simulink model "clamped_plate_NASTRAN_aug"  (R2025b)
settings: Solver=VariableStepAuto  StartTime=0.0  StopTime=10  RelTol=1e-3
libraries: RCTblocks x1
settings Model: Creator=f.sanfedino  LastModifiedBy=andre
settings SolverCC: AlgebraicLoopSolver=TrustRegion
settings DataIOCC: ReturnWorkspaceOutputs=off
settings DebuggingCC: UnconnectedInputMsg=warning  UnconnectedOutputMsg=warning  UnconnectedLineMsg=warning
settings ModelReferenceCC: EnableRefExpFcnMdlSchedulingChecks=on
settings RTWCC: GPUComputeCapability=3.5  DLArmComputeVersion=19.05

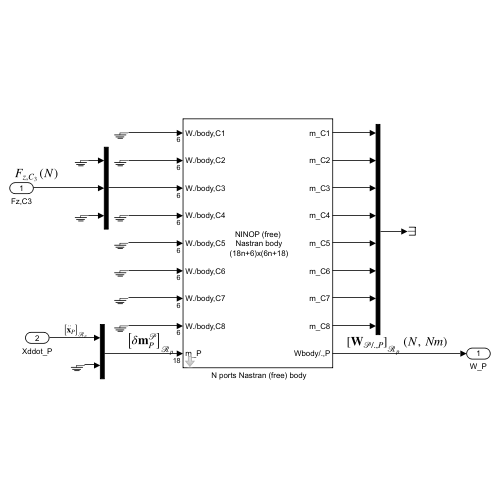
[thumbnail: Simulink's stored preview of the top-level diagram]
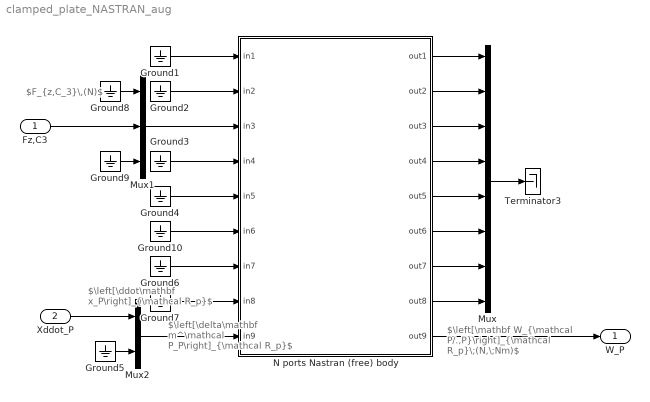
== system clamped_plate_NASTRAN_aug ==
  note: $F_{z,C_3}\,(N)$
  note: $\left[\mathbf W_{\mathcal P/.,P}\right]_{\mathcal R_p}\;(N,\;Nm)$
  note: $\left[\delta\mathbf m^\mathcal P_P\right]_{\mathcal R_p}$
  note: $\left[\ddot\mathbf x_P\right]_{\mathcal R_p}$
  Fz,C3 : Inport
  Xddot_P : Inport  Port=2
  " N ports Nastran (free) body" : Subsystem  mask(NINOP Model of a Nastran body){fbdf='fbdf_plate', ff06='ff06_plate', P_gp=56, C_gp=[1;6;11;61;66;111;116;121], nf=20, Xi=0.001, free=off, uw_var=0, Nflex_w=0, uls_var=5, Nflex_LP=0, uev_var=0, Nflex_EV=0}
      mask prompts: fbdf "Name of the .bdf file (without extension)"; ff06 "Name of the .f06 file (without extension)"; P_gp "Node number corresponding to the point P (connection with parent body)"; C_gp "Node numbers corresponding to the points C (connections with child bodies)"; nf "Number of modes to be considered"; Xi "Common damping ratio"; free "Free body at P"; uw_var "uncertainties (%)"; Nflex_w "number of flexible modes (integer)"; uls_var "uncertainties (%)"; Nflex_LP "number of flexible modes (integer)"; uev_var "uncertainties (%)"; Nflex_EV "number of flexible modes (integer)"
      mask help:
      | NINOP (18n+6)x(6n+18) model of a flexible body at points C (connection point with the child  bodies) and point P (connection point with a parent body).
      | * 18nx6n transfer between the wrench applied to this body at the child points C  and motion vectors at these points
      | * 6x18 transfer between the motion vector at the "parent" point P  and the wrench applied by this body at this point
      | The model is expressed In the (inherit) body frame.
      |
      | Model is built from  the data provided by Patran/Nastran analysis output files.
      | Uncertainties can be added to the main parameters.
      |
      | RK: The last channel associated to parent port P can be inverted to free the body at the point P. In that case, 6 rigid modes (12 integrators) are added in the model to output the motion vector at the point P and the model becomes 18(n+1)x6(n+1).
      mask init:
      | n = length(C_gp);
      | NastranBodyNPortAugFree
      mask Help: web('DocNPortNastranBody.html','-browser')
      mask DialogControl Container2 Prompt: Main parameters
      mask DialogControl Container6 Prompt: Parametric uncertainties:
      mask DialogControl Container8 Prompt: Frequencies
      mask DialogControl Control18 Prompt: A common relative uncertainty (%) on the first flexible mode frequencies can be added (uncertainties can be changed later)
      mask DialogControl Control3 Prompt: The uncertain frequency is named: 'w_name_i' where:
      mask DialogControl Control4 Prompt: * 'name' is the current block name (reduced to its alphanumeric characters).
      mask DialogControl Control17 Prompt: * 'i' is the flexible mode number (increasing frequency order)
      mask DialogControl Container9 Prompt: Modal participation factors
      mask DialogControl Control20 Prompt: A common relative uncertainty (%) on the modal participation factors of the first flexible modes can be added (uncertainties can be changed later)
      mask DialogControl Control6 Prompt: The uncertain modal participation factor is named: 'LP_name_iXX' where:
      mask DialogControl Control7 Prompt: *  'name' is the current block name (reduced to its alphanumeric characters),
      mask DialogControl Control8 Prompt: * 'i' is the flexible mode number (increasing frequency order),
      mask DialogControl Control9 Prompt: * 'XX' = 'Tx', 'Ty', 'Tz', 'Rx', 'Ry', 'Rz'.
      mask DialogControl Container10 Prompt: Modal shapes
      mask DialogControl Control21 Prompt: A common relative uncertainty (%) on each eigen vector components at points C for the first flexible modes can be added (uncertainties can be changed later)
      mask DialogControl Control16 Prompt: WARNING: can generate very long process time !!
      mask DialogControl Control11 Prompt: The uncertain component is named: "EV_name_Cj_iXX' where:
      mask DialogControl Control12 Prompt: * 'name' is the current block name (reduced to its alphanumeric characters).
      mask DialogControl Control13 Prompt: * 'j' is the point C number,
      mask DialogControl Control14 Prompt: * 'i' is the flexible mode number (increasing frequency order),
      mask DialogControl Control15 Prompt: * 'XX' = 'Tx', 'Ty', 'Tz', 'Rx', 'Ry', 'Rz'.
      mask Display:
      | if free
      |     disp('NINOP (free)\n Nastran body\n 18(n+1)x6(n+1)')
      | else
      |     disp('NINOP (free)\n Nastran body\n (18n+6)x(6n+18)')
      | end
      | 
      | for ii=1:n
      |         port_label('input', ii,['W./body,C',num2str(ii)])
      |         port_label('output',ii,['m_C',num2str(ii)])
      | end
      | 
      | if free
      |     port_label('input', n+1,'W./body,P')
      |     port_label('output',n+1,'m_P')
      | else
      |     port_label('input', n+1,'m_P')
      |     port_label('output',n+1,'Wbody/.,P')
      | end
  Ground{1..10} (10 alike) : Ground
  Mux : Mux  Inputs=18*ones(1,8)
  Mux1 : Mux  Inputs=[2 1 3]
  Mux2 : Mux  Inputs=[6 12]
  Terminator3 : Terminator
  W_P : Outport
  wires:
  Mux2/1 -> " N ports Nastran (free) body"/9(in9)
  Ground1/1 -> " N ports Nastran (free) body"/1(in1)
  Ground2/1 -> " N ports Nastran (free) body"/2(in2)
  Ground4/1 -> " N ports Nastran (free) body"/5(in5)
  Ground3/1 -> " N ports Nastran (free) body"/4(in4)
  Ground6/1 -> " N ports Nastran (free) body"/7(in7)
  Ground7/1 -> " N ports Nastran (free) body"/8(in8)
  " N ports Nastran (free) body"/1(out1) -> Mux/1
  " N ports Nastran (free) body"/2(out2) -> Mux/2
  " N ports Nastran (free) body"/3(out3) -> Mux/3
  " N ports Nastran (free) body"/4(out4) -> Mux/4
  " N ports Nastran (free) body"/5(out5) -> Mux/5
  " N ports Nastran (free) body"/6(out6) -> Mux/6
  " N ports Nastran (free) body"/7(out7) -> Mux/7
  " N ports Nastran (free) body"/8(out8) -> Mux/8
  " N ports Nastran (free) body"/9(out9) -> W_P/1
  Mux1/1 -> " N ports Nastran (free) body"/3(in3)
  Ground8/1 -> Mux1/1
  Ground9/1 -> Mux1/3
  Ground10/1 -> " N ports Nastran (free) body"/6(in6)
  Fz,C3/1 -> Mux1/2
  Mux/1 -> Terminator3/1
  Xddot_P/1 -> Mux2/1
  Ground5/1 -> Mux2/2

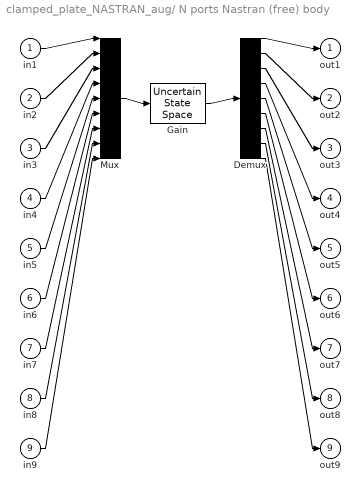
== system clamped_plate_NASTRAN_aug/ N ports Nastran (free) body ==
  in1 : Inport  PortDimensions=6
  in2 : Inport  Port=2  PortDimensions=6
  in3 : Inport  Port=3  PortDimensions=6
  in4 : Inport  Port=4  PortDimensions=6
  in5 : Inport  Port=5  PortDimensions=6
  in6 : Inport  Port=6  PortDimensions=6
  in7 : Inport  Port=7  PortDimensions=6
  in8 : Inport  Port=8  PortDimensions=6
  in9 : Inport  Port=9  PortDimensions=18
  Demux : Demux  Outputs=[18 18 18 18 18 18 18 18 6]
  Gain : RCTblocks/Uncertain State Space  Tag=USS  USystem=Mdyn  UValue=[]  X0=[]  uX0=[]
  Mux : Mux  Inputs=[6 6 6 6 6 6 6 6 18]
  out1 : Outport
  out2 : Outport  Port=2
  out3 : Outport  Port=3
  out4 : Outport  Port=4
  out5 : Outport  Port=5
  out6 : Outport  Port=6
  out7 : Outport  Port=7
  out8 : Outport  Port=8
  out9 : Outport  Port=9
  wires:
  Mux/1 -> Gain/1
  Gain/1 -> Demux/1
  in1/1 -> Mux/1
  Demux/1 -> out1/1
  in2/1 -> Mux/2
  Demux/2 -> out2/1
  in3/1 -> Mux/3
  Demux/3 -> out3/1
  in4/1 -> Mux/4
  Demux/4 -> out4/1
  in5/1 -> Mux/5
  Demux/5 -> out5/1
  in6/1 -> Mux/6
  Demux/6 -> out6/1
  in7/1 -> Mux/7
  Demux/7 -> out7/1
  in8/1 -> Mux/8
  Demux/8 -> out8/1
  in9/1 -> Mux/9
  Demux/9 -> out9/1
